simulink model "Cobot600_PathFeedback"  (R2024b)
settings: Solver=FixedStepAuto  StartTime=0.0  StopTime=stopsim  FixedStep=0.5  RelTol=1e-3
values from neighbouring files (symbols this model uses):
  x_start = X(1)    [MyCobotPro_PathPlanning.m]
  y_start = Y(1)    [MyCobotPro_PathPlanning.m]
libraries: robotcorelib x1, robotmaniplib x1
settings Model: Creator=almas  LastModifiedBy=almas

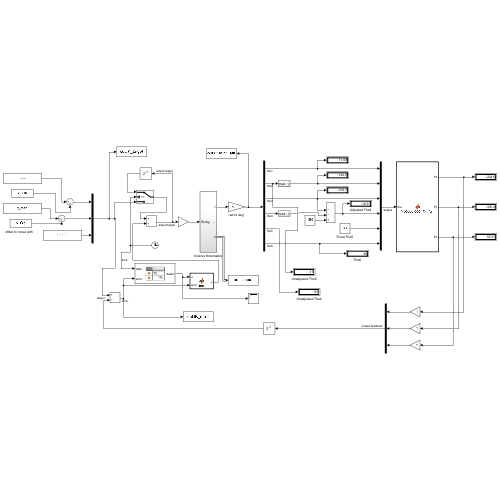
[thumbnail: Simulink's stored preview of the top-level diagram]
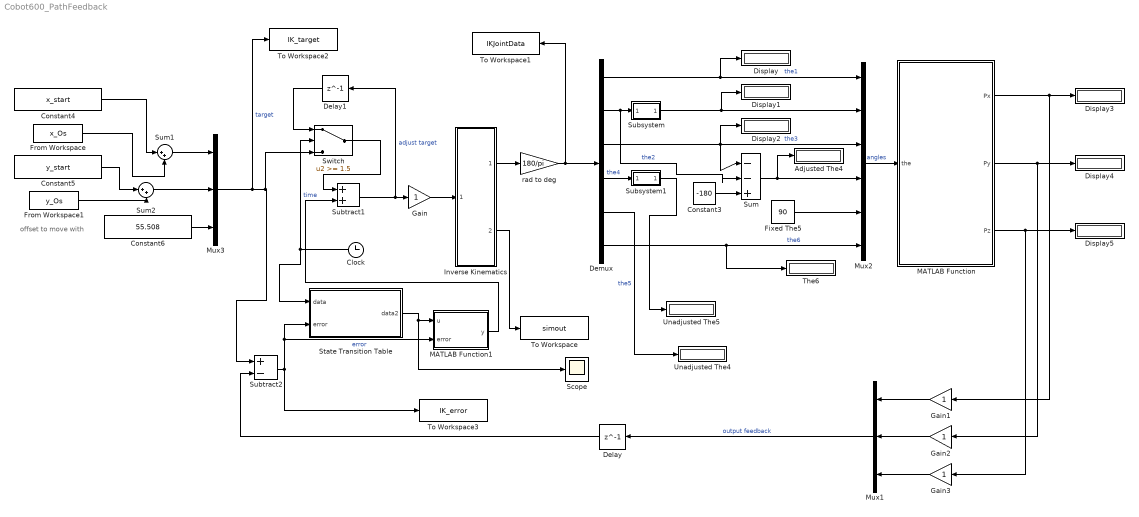
== system Cobot600_PathFeedback ==
  note: offset to move with
  Adjusted The4 : Display
  Clock : Clock
  Constant3 : Constant  Value=-180
  Constant4 : Constant  Value=x_start  SampleTime=0.5
  Constant5 : Constant  Value=y_start  SampleTime=0.5
  Constant6 : Constant  Value=55.508  SampleTime=0.5
  Delay : Delay  DelayLength=1
  Delay1 : Delay  DelayLength=1
  Demux : Demux  Outputs=6
  Display{,1..5} (6 alike) : Display
  Fixed The5 : Constant  Value=90
  From Workspace : FromWorkspace  VariableName=x_Os  SampleTime=0.5  Interpolate=off  OutputAfterFinalValue=Holding final value
  From Workspace1 : FromWorkspace  VariableName=y_Os  SampleTime=0.5  Interpolate=off  OutputAfterFinalValue=Holding final value
  Gain{,1..3} (4 alike) : Gain
  Inverse Kinematics : Subsystem
  MATLAB Function : MATLAB Function  TreatAsAtomicUnit=on
  MATLAB Function1 : MATLAB Function  TreatAsAtomicUnit=on
  Mux1 : Mux  Inputs=3
  Mux2 : Mux  Inputs=6
  Mux3 : Mux  Inputs=3
  Scope : Scope
  State Transition Table : State Transition Table  TreatAsAtomicUnit=on
      settings: PortSchema="{\"entries\":[{\"content\":{\"sides\":[{\"content\":{\"connectorIds\":[\"In2\",\"In1\"]},\"type\":\"ConnectorPlacement.EquallySpacedRectSide\",\"uuid\":\"11c50549-ecbc-46f3-8ae4-b1d7b65dda60\"},{\"content\":{\"connectorIds\":[\"Out1\"],\"side\":\"RIGHT\"},\"type\":\"ConnectorPlacement.EquallySpacedRectSide\",\"uuid\":\"8c490834-a0a3-44e7-815c-33f6e1acb8e7\"},{\"content\":{\"side\":\"TOP\"},\"type\":\"ConnectorPlacement.EquallySpacedRectSide\",\"uuid\":\"740cc173-e692-47d5-80e1-49ea57bd09db\"},{\"content\":{\"side\":\"BOTTOM\"},\"type\":\"ConnectorPlacement.EquallySpacedRectSide\",\"uuid\":\"26f1aca0-c1b6-4773-8aea-3cd547beedd7\"}]},\"type\":\"ConnectorPlacement.EquallySpacedConnector\",\"uuid\":\"86b59f75-8780-4864-be1e-7919a6aa9c61\"}],\"packageUris\":[\"http://schema.mathworks.com/mf0/Connector/R2020b\"],\"version\":\"1.0\"}"
  Subsystem : Subsystem
  Subsystem1 : Subsystem
  Subtract1 : Sum
  Subtract2 : Sum  Inputs=+-
  Sum : Sum  Inputs=|--+
  Sum1 : Sum  Inputs=|++
  Sum2 : Sum  Inputs=|++
  Switch : Switch  Threshold=1.5  SaturateOnIntegerOverflow=off  InputSameDT=off
  The6 : Display
  To Workspace : ToWorkspace  VariableName=simout  SaveFormat=Timeseries  SampleTime=-1
  To Workspace1 : ToWorkspace  VariableName=IKJointData  SampleTime=-1
      settings: Save2DSignal=2-D array (concatenate along first dimension)
  To Workspace2 : ToWorkspace  VariableName=IK_target  SampleTime=-1
      settings: Save2DSignal=2-D array (concatenate along first dimension)
  To Workspace3 : ToWorkspace  VariableName=IK_error  SampleTime=-1
      settings: Save2DSignal=2-D array (concatenate along first dimension)
  Unadjusted The4 : Display
  Unadjusted The5 : Display
  "rad to deg " : Gain  Gain=180/pi
  wires:
  Inverse Kinematics/2(Out2) -> To Workspace/1
  Inverse Kinematics/1(Out1) -> "rad to deg "/1
  Demux/1 -> Display/1, Mux2/1  "the1"
  Demux/5 -> Unadjusted The4/1  "the5"
  Demux/6 -> The6/1, Mux2/6  "the6"
  Demux/3 -> Display2/1, Mux2/3, Sum/1  "the3"
  Mux3/1 -> To Workspace2/1, Switch/3, Subtract2/1  "target"
  "rad to deg "/1 -> To Workspace1/1, Demux/1
  Subsystem/1(Out1) -> Display1/1, Mux2/2
  Demux/2 -> Sum/2, Subsystem/1(the2)  "the2"
  Subsystem1/1(Out1) -> Unadjusted The5/1
  Demux/4 -> Subsystem1/1(the4)  "the4"
  Constant3/1 -> Sum/3
  Sum/1 -> Mux2/4, Adjusted The4/1
  Fixed The5/1 -> Mux2/5
  Gain/1 -> Inverse Kinematics/1(Config)
  MATLAB Function/1(Px) -> Gain1/1, Display3/1
  MATLAB Function/3(Pz) -> Gain3/1, Display5/1
  MATLAB Function/2(Py) -> Gain2/1, Display4/1
  Gain1/1 -> Mux1/1
  Gain2/1 -> Mux1/2
  Gain3/1 -> Mux1/3
  Clock/1 -> State Transition Table/2(data), Switch/2  "time"
  Subtract2/1 -> MATLAB Function1/2(error), State Transition Table/1(error), To Workspace3/1  "error"
  Subtract1/1 -> Delay1/1, Gain/1  "adjust target"
  Switch/1 -> Subtract1/1
  Delay1/1 -> Switch/1
  Mux1/1 -> Delay/1  "output feedback"
  Delay/1 -> Subtract2/2
  State Transition Table/1(data2) -> Scope/1, MATLAB Function1/1(u)
  MATLAB Function1/1(y) -> Subtract1/2
  Mux2/1 -> MATLAB Function/1(the)  "angles"
  Constant6/1 -> Mux3/3
  Constant4/1 -> Sum1/1
  Sum1/1 -> Mux3/1
  From Workspace/1 -> Sum1/2
  Constant5/1 -> Sum2/1
  From Workspace1/1 -> Sum2/2
  Sum2/1 -> Mux3/2

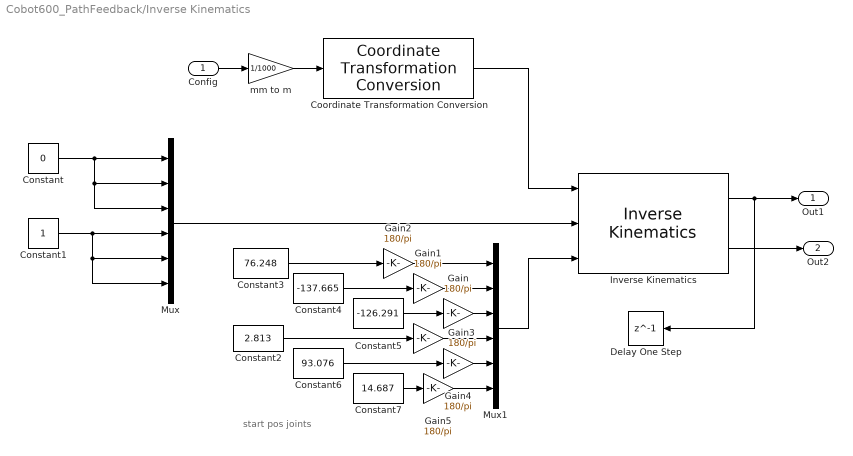
== system Cobot600_PathFeedback/Inverse Kinematics ==
  note: start pos joints
  Config : Inport
  Constant : Constant  Value=0
  Constant1 : Constant
  Constant2 : Constant  Value=2.813
  Constant3 : Constant  Value=76.248
  Constant4 : Constant  Value=-137.665
  Constant5 : Constant  Value=-126.291
  Constant6 : Constant  Value=93.076
  Constant7 : Constant  Value=14.687
  Coordinate Transformation Conversion : robotcorelib/Coordinate Transformation Conversion  InputRepresentation=Translation Vector  InputEulerSequence=ZYX  ShowTrVecInputPort=on  OutputRepresentation=Homogeneous Transformation  OutputEulerSequence=ZYX  ShowTrVecOutputPort=on  SimulateUsing=Interpreted execution
  Delay One Step : Delay  DelayLength=1
  Gain{,1..5} (6 alike) : Gain  Gain=180/pi
  Inverse Kinematics : robotmaniplib/Inverse Kinematics  RigidBodyTree=myCobotBU  EndEffector=Body6  ShowInfo=on  SolverName=BFGS Gradient Projection  EnforceJointLimits=on  MaxIterations=1500  MaxTime=10  GradientTolerance=1e-7  SolutionTolerance=1e-6  StepTolerance=1e-14  ErrorChangeTolerance=1e-12  UseErrorDamping=on  DampingBias=0.0025  SimulateUsing=Interpreted execution
  Mux : Mux  Inputs=6
  Mux1 : Mux  Inputs=6
  mm to m : Gain  Gain=1/1000
  Out1 : Outport
  Out2 : Outport  Port=2
  wires:
  Inverse Kinematics/1 -> Delay One Step/1, Out1/1
  Config/1 -> mm to m/1
  Coordinate Transformation Conversion/1 -> Inverse Kinematics/1
  Inverse Kinematics/2 -> Out2/1
  Mux/1 -> Inverse Kinematics/2
  Constant/1 -> Mux/2, Mux/3, Mux/1
  Constant1/1 -> Mux/6, Mux/5, Mux/4
  mm to m/1 -> Coordinate Transformation Conversion/1
  Constant3/1 -> Gain2/1
  Constant4/1 -> Gain1/1
  Constant5/1 -> Gain/1
  Gain/1 -> Mux1/3
  Gain2/1 -> Mux1/1
  Gain1/1 -> Mux1/2
  Constant2/1 -> Gain3/1
  Constant7/1 -> Gain5/1
  Constant6/1 -> Gain4/1
  Gain3/1 -> Mux1/4
  Gain4/1 -> Mux1/5
  Gain5/1 -> Mux1/6
  Mux1/1 -> Inverse Kinematics/3

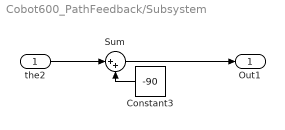
== system Cobot600_PathFeedback/Subsystem ==
  the2 : Inport
  Constant3 : Constant  Value=-90
  Sum : Sum  Inputs=|++
  Out1 : Outport
  wires:
  Constant3/1 -> Sum/2
  the2/1 -> Sum/1
  Sum/1 -> Out1/1

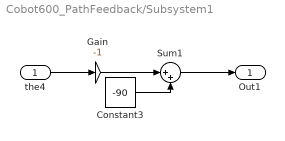
== system Cobot600_PathFeedback/Subsystem1 ==
  the4 : Inport
  Constant3 : Constant  Value=-90
  Gain : Gain  Gain=-1
  Sum1 : Sum  Inputs=|++
  Out1 : Outport
  wires:
  Gain/1 -> Sum1/1
  Constant3/1 -> Sum1/2
  the4/1 -> Gain/1
  Sum1/1 -> Out1/1

== matlab function Cobot600_PathFeedback/MATLAB Function1 ==
  data: u input; y output; error input
function y = fcn(u, error)
if sum(abs(error))/3 < 1.5
    y = error;
else 
    y = u;
end

== matlab function Cobot600_PathFeedback/MATLAB Function ==
  data: the input; Px output; Py output; Pz output
function [Px, Py, Pz] = MyCobot600_FK_fun(the)
    % Cobot Values 
    a1 = 210;
    a2 = 250;
    a3 = 250;
    a4 = 109.5;
    a5 = 107; 
    a6 = 76.2;
    % deg to rad conversion 
    t1 = the(1)*pi/180; t2 = the(2)*pi/180; t3 = the(3)*pi/180; t4 = the(4)*pi/180; t5 = the(5)*pi/180; 
    %t6 = t6*pi/180;
    
    % X/Y/Z position from Transformation Matrix
    Px = a2*cos(t1)*cos(t2) - a4*sin(t1) - a6*cos(t5)*sin(t1) - a5*sin(t2 + t3 + t4)*cos(t1) + a3*cos(t1)*cos(t2)*cos(t3) - a3*cos(t1)*sin(t2)*sin(t3) + a6*cos(t2 + t3 + t4)*cos(t1)*sin(t5);   
    Py = a6*(cos(t1)*cos(t5) + cos(t2 + t3 + t4)*sin(t1)*sin(t5)) + a4*cos(t1) + a2*cos(t2)*sin(t1) - a5*sin(t2 + t3 + t4)*sin(t1) + a3*cos(t2)*cos(t3)*sin(t1) - a3*sin(t1)*sin(t2)*sin(t3);
    Pz = a1 + a5*(sin(t2 + t3)*sin(t4) - cos(t2 + t3)*cos(t4)) - a3*sin(t2 + t3) - a2*sin(t2) - a6*sin(t5)*(cos(t2 + t3)*sin(t4) + sin(t2 + t3)*cos(t4));

== stateflow chart Cobot600_PathFeedback/State Transition Table ==
  state state1
    data2 = [0;0;0];
  state state2
    data2 = error;
  state state3
    data2 = error*0.5;
  state state4
    data2 = [0; 0; 0];
  (default) -> state1
  state1 -> state2 : [data > 0]
  (junction 45) -> state2
  state2 -> (junction 35) [order 1] : [sum(abs(error))/3 < 0.5]
  (junction 47) -> (junction 45)
  (junction 35) -> (junction 33)
  state2 -> state3 [order 2] : [sum(abs(error))/3 > 20]
  state3 -> state2 : [sum(abs(error))/3 <= 20]
  state4 -> (junction 47) : [sum(abs(error))/3 > 2.5]
  (junction 33) -> state4
  data: error input; data input; data2 output
